simulink model "Main"  (R2025b)
settings: Solver=ode4  StartTime=0.0  StopTime=40  FixedStep=0.01  RelTol=1e-3
undefined symbols (not defined in the file): d_geo, DiscIntNeverNeededParam, t_geo, t_rotation, t_velocity
settings Model: DataDictionary=Main_data.sldd  VariantFading=off  Creator=mauro  LastModifiedBy=mauro

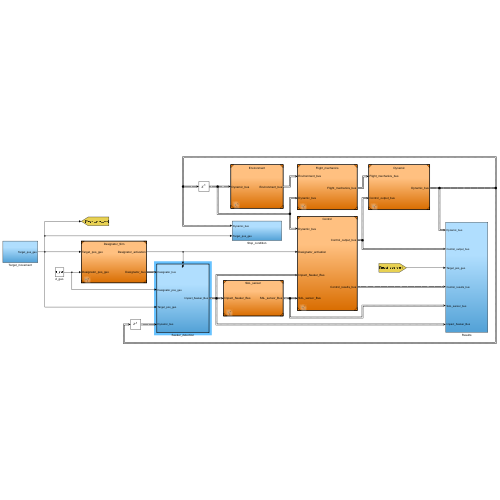
[thumbnail: Simulink's stored preview of the top-level diagram]
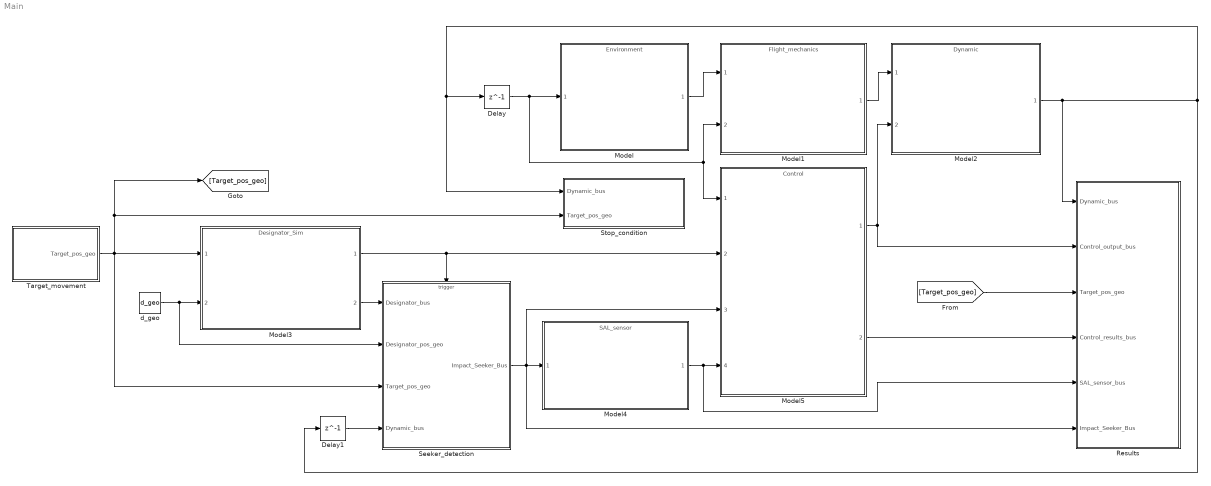
== system Main ==
  Delay : Delay  DelayLength=1  InitialCondition=0
  Delay1 : Delay  DelayLength=1  InitialCondition=0
  Model : ModelReference  ModelNameDialog=Environment.slx  SimulationMode=Normal  ModelReferenceVersion=1.30
  Model1 : ModelReference  ModelNameDialog=Flight_mechanics.slx  SimulationMode=Normal  ModelReferenceVersion=1.31
  Model2 : ModelReference  ModelNameDialog=Dynamic.slx  SimulationMode=Normal  ModelReferenceVersion=1.41
  Model3 : ModelReference  ModelNameDialog=Designator_Sim.slx  SimulationMode=Normal  ModelReferenceVersion=1.21
  Model4 : ModelReference  ModelNameDialog=SAL_sensor.slx  SimulationMode=Normal  ModelReferenceVersion=1.37
  Model5 : ModelReference  ModelNameDialog=Control.slx  SimulationMode=Normal  ModelReferenceVersion=1.50
  Results : Subsystem
  Seeker_detection : Subsystem
  Stop_condition : Subsystem
  Target_movement : Subsystem
  d_geo : Constant  Value=d_geo
  wires:
  Model1/1 -> Model2/1
  Model/1 -> Model1/1
  Model2/1 -> Delay1/1, Stop_condition/1(Dynamic_bus), Delay/1, Results/1(Dynamic_bus)
  Delay/1 -> Model5/1, Model1/2, Model/1
  Seeker_detection/1(Impact_Seeker_Bus) -> Model5/3, Results/6(Impact_Seeker_Bus), Model4/1
  Delay1/1 -> Seeker_detection/4(Dynamic_bus)
  Model3/2 -> Seeker_detection/1(Designator_bus)
  d_geo/1 -> Seeker_detection/2(Designator_pos_geo), Model3/2
  Model5/1 -> Results/2(Control_output_bus), Model2/2
  Model4/1 -> Results/5(SAL_sensor_bus), Model5/4
  Model3/1 -> Seeker_detection/Trigger, Model5/2
  [Target_pos_geo] -> Results/3(Target_pos_geo)
  Model5/2 -> Results/4(Control_results_bus)
  Target_movement/1(Target_pos_geo) -> Stop_condition/2(Target_pos_geo), [Target_pos_geo], Seeker_detection/3(Target_pos_geo), Model3/1

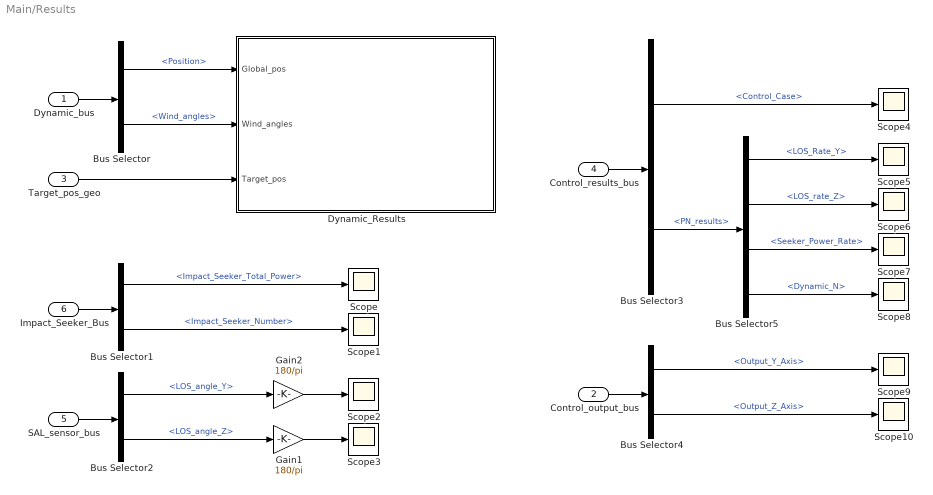
== system Main/Results ==
  Dynamic_bus : Inport  OutDataTypeStr=Bus: Dynamic_bus
  Control_output_bus : Inport  Port=2
  Target_pos_geo : Inport  Port=3
  Control_results_bus : Inport  Port=4
  SAL_sensor_bus : Inport  Port=5
  Impact_Seeker_Bus : Inport  Port=6
  Bus Selector : BusSelector  OutputSignals=Position,Wind_angles
  Bus Selector1 : BusSelector  OutputSignals=Impact_Seeker_Total_Power,Impact_Seeker_Number
  Bus Selector2 : BusSelector  OutputSignals=LOS_angle_Y,LOS_angle_Z
  Bus Selector3 : BusSelector  OutputSignals=Control_Case,PN_results
  Bus Selector4 : BusSelector  OutputSignals=Output_Y_Axis,Output_Z_Axis
  Bus Selector5 : BusSelector  OutputSignals=LOS_Rate_Y,LOS_rate_Z,Seeker_Power_Rate,Dynamic_N
  Dynamic_Results : Subsystem
  Gain1 : Gain  Gain=180/pi
  Gain2 : Gain  Gain=180/pi
  Scope{,1..10} (11 alike) : Scope
      Scope settings: ActiveDisplayYMinimum=-0.0017009499425087375  ActiveDisplayYMaximum=0.015308549482578641
      Scope1 settings: ActiveDisplayYMinimum=-4068.8424899316433  ActiveDisplayYMaximum=14541.688244827959  DataLoggingVariableName=ScopeData4
      Scope10 settings: ActiveDisplayYMinimum=-538.883824388517  ActiveDisplayYMaximum=718.00642075117651  DataLoggingVariableName=ScopeData13
      Scope2 settings: ActiveDisplayYMinimum=-1  ActiveDisplayYMaximum=1  DataLoggingVariableName=ScopeData5
      Scope3 settings: ActiveDisplayYMinimum=-9.0449990210259017  ActiveDisplayYMaximum=11.160194306089778  DataLoggingVariableName=ScopeData6
      Scope4 settings: ActiveDisplayYMinimum=-0.24999999999999994  ActiveDisplayYMaximum=2.25  DataLoggingVariableName=ScopeData7
      Scope5 settings: ActiveDisplayYMinimum=-0.00011873889811281793  ActiveDisplayYMaximum=0.00016852439541605621  DataLoggingVariableName=ScopeData8
      Scope6 settings: ActiveDisplayYMinimum=-0.65509945125026314  ActiveDisplayYMaximum=0.56583480808345421  DataLoggingVariableName=ScopeData9
      Scope7 settings: ActiveDisplayYMinimum=-0.26313284982804819  ActiveDisplayYMaximum=0.28806425796157659  DataLoggingVariableName=ScopeData10
      Scope8 settings: ActiveDisplayYMinimum=-0.25636599959653461  ActiveDisplayYMaximum=13.637920041276896  DataLoggingVariableName=ScopeData11
      Scope9 settings: ActiveDisplayYMinimum=-1  ActiveDisplayYMaximum=1  DataLoggingVariableName=ScopeData12
  wires:
  Dynamic_bus/1 -> Bus Selector/1
  Target_pos_geo/1 -> Dynamic_Results/3(Target_pos)
  Bus Selector/1 -> Dynamic_Results/1(Global_pos)  "<Position>"
  Bus Selector/2 -> Dynamic_Results/2(Wind_angles)  "<Wind_angles>"
  Impact_Seeker_Bus/1 -> Bus Selector1/1
  Bus Selector1/1 -> Scope/1  "<Impact_Seeker_Total_Power>"
  Bus Selector1/2 -> Scope1/1  "<Impact_Seeker_Number>"
  SAL_sensor_bus/1 -> Bus Selector2/1
  Bus Selector2/1 -> Gain2/1  "<LOS_angle_Y>"
  Bus Selector2/2 -> Gain1/1  "<LOS_angle_Z>"
  Control_results_bus/1 -> Bus Selector3/1
  Control_output_bus/1 -> Bus Selector4/1
  Bus Selector3/2 -> Bus Selector5/1  "<PN_results>"
  Bus Selector3/1 -> Scope4/1  "<Control_Case>"
  Bus Selector5/1 -> Scope5/1  "<LOS_Rate_Y>"
  Bus Selector5/2 -> Scope6/1  "<LOS_rate_Z>"
  Bus Selector5/4 -> Scope8/1  "<Dynamic_N>"
  Bus Selector5/3 -> Scope7/1  "<Seeker_Power_Rate>"
  Bus Selector4/1 -> Scope9/1  "<Output_Y_Axis>"
  Gain2/1 -> Scope2/1
  Gain1/1 -> Scope3/1
  Bus Selector4/2 -> Scope10/1  "<Output_Z_Axis>"

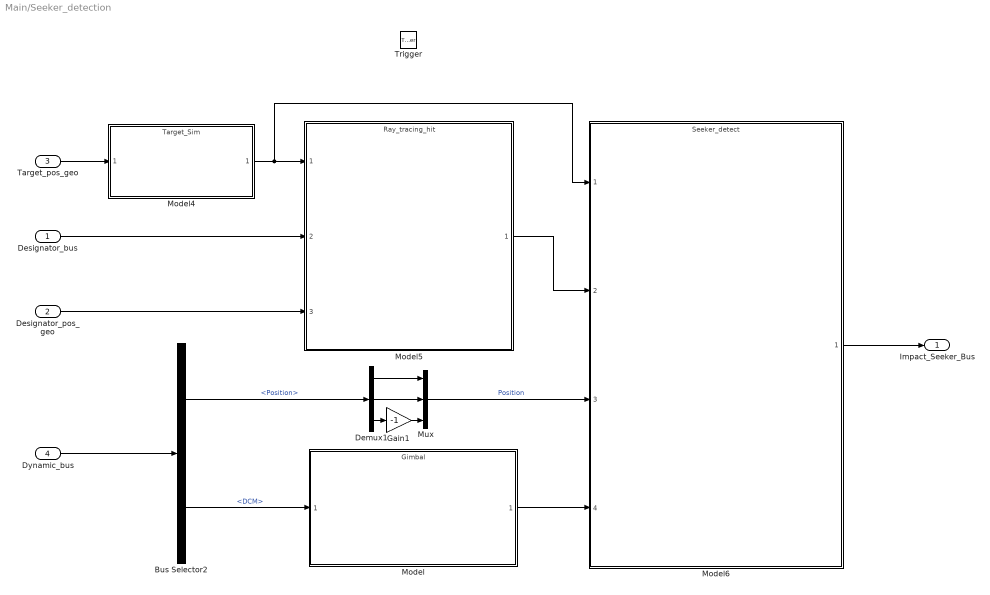
== system Main/Seeker_detection ==
  Designator_bus : Inport  OutDataTypeStr=Bus: Designator_bus
  Designator_pos_geo : Inport  Port=2
  Target_pos_geo : Inport  Port=3
  Dynamic_bus : Inport  Port=4  OutDataTypeStr=Bus: Dynamic_bus
  Trigger : TriggerPort  VariantControl=(inherit)  PortDimensions=1
  Bus Selector2 : BusSelector  OutputSignals=Position,DCM
  Demux1 : Demux  Outputs=3
  Gain1 : Gain  Gain=-1
  Model : ModelReference  ModelNameDialog=Gimbal.slx  SimulationMode=Normal  ModelReferenceVersion=1.16
  Model4 : ModelReference  ModelNameDialog=Target_Sim.slx  SimulationMode=Normal  ModelReferenceVersion=1.19
  Model5 : ModelReference  ModelNameDialog=Ray_tracing_hit.slx  SimulationMode=Normal  ModelReferenceVersion=1.26
  Model6 : ModelReference  ModelNameDialog=Seeker_detect.slx  SimulationMode=Normal  ModelReferenceVersion=1.23
  Mux : Mux  Inputs=3
  Impact_Seeker_Bus : Outport  OutDataTypeStr=Bus: Impact_Seeker_Bus
  wires:
  Model6/1 -> Impact_Seeker_Bus/1
  Model5/1 -> Model6/2
  Dynamic_bus/1 -> Bus Selector2/1
  Model4/1 -> Model6/1, Model5/1
  Target_pos_geo/1 -> Model4/1
  Designator_pos_geo/1 -> Model5/3
  Designator_bus/1 -> Model5/2
  Bus Selector2/1 -> Demux1/1  "<Position>"
  Bus Selector2/2 -> Model/1  "<DCM>"
  Model/1 -> Model6/4
  Demux1/1 -> Mux/1
  Demux1/3 -> Gain1/1
  Demux1/2 -> Mux/2
  Gain1/1 -> Mux/3
  Mux/1 -> Model6/3  "Position"

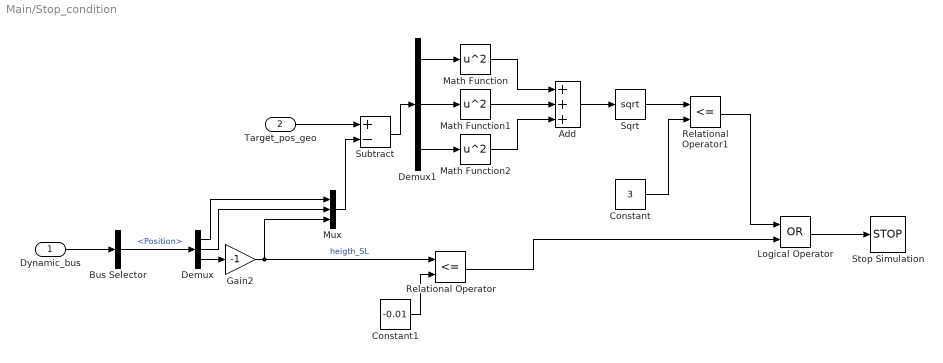
== system Main/Stop_condition ==
  Dynamic_bus : Inport  OutDataTypeStr=Bus: Dynamic_bus
  Target_pos_geo : Inport  Port=2
  Add : Sum  Inputs=+++
  Bus Selector : BusSelector  OutputSignals=Position
  Constant : Constant  Value=3
  Constant1 : Constant  Value=-0.01
  Demux : Demux  Outputs=3
  Demux1 : Demux  Outputs=3
  Gain2 : Gain  Gain=-1
  Logical Operator : Logic  Operator=OR  AllPortsSameDT=off  OutDataTypeStr=boolean
  Math Function : Math  Operator=square
  Math Function1 : Math  Operator=square
  Math Function2 : Math  Operator=square
  Mux : Mux  Inputs=3
  Relational Operator : RelationalOperator  Operator=<=  OutDataTypeStr=boolean  RndMeth=Simplest  InputSameDT=off
  Relational Operator1 : RelationalOperator  Operator=<=  OutDataTypeStr=boolean  RndMeth=Simplest  InputSameDT=off
  Sqrt : Sqrt
  Stop Simulation : Stop
  Subtract : Sum  Inputs=+-
  wires:
  Constant1/1 -> Relational Operator/2
  Dynamic_bus/1 -> Bus Selector/1
  Bus Selector/1 -> Demux/1  "<Position>"
  Demux/3 -> Gain2/1
  Gain2/1 -> Mux/3, Relational Operator/1  "heigth_SL"
  Logical Operator/1 -> Stop Simulation/1
  Relational Operator/1 -> Logical Operator/2
  Demux/1 -> Mux/1
  Demux/2 -> Mux/2
  Target_pos_geo/1 -> Subtract/1
  Mux/1 -> Subtract/2
  Subtract/1 -> Demux1/1
  Constant/1 -> Relational Operator1/2
  Demux1/1 -> Math Function/1
  Demux1/2 -> Math Function1/1
  Demux1/3 -> Math Function2/1
  Math Function1/1 -> Add/2
  Math Function/1 -> Add/1
  Math Function2/1 -> Add/3
  Add/1 -> Sqrt/1
  Sqrt/1 -> Relational Operator1/1
  Relational Operator1/1 -> Logical Operator/1

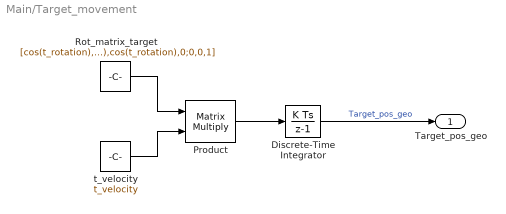
== system Main/Target_movement ==
  Discrete-Time Integrator : DiscreteIntegrator  InitialCondition=t_geo  SampleTime=-1  ICPrevOutput=DiscIntNeverNeededParam  ICPrevScaledInput=DiscIntNeverNeededParam
  Product : Product  Multiplication=Matrix(*)
  Rot_matrix_target : Constant  Value=[cos(t_rotation),-sin(t_rotation),0;sin(t_rotation),cos(t_rotation),0;0,0,1]
  t_velocity : Constant  Value=t_velocity
  Target_pos_geo : Outport
  wires:
  Rot_matrix_target/1 -> Product/1
  Product/1 -> Discrete-Time Integrator/1
  t_velocity/1 -> Product/2
  Discrete-Time Integrator/1 -> Target_pos_geo/1  "Target_pos_geo"

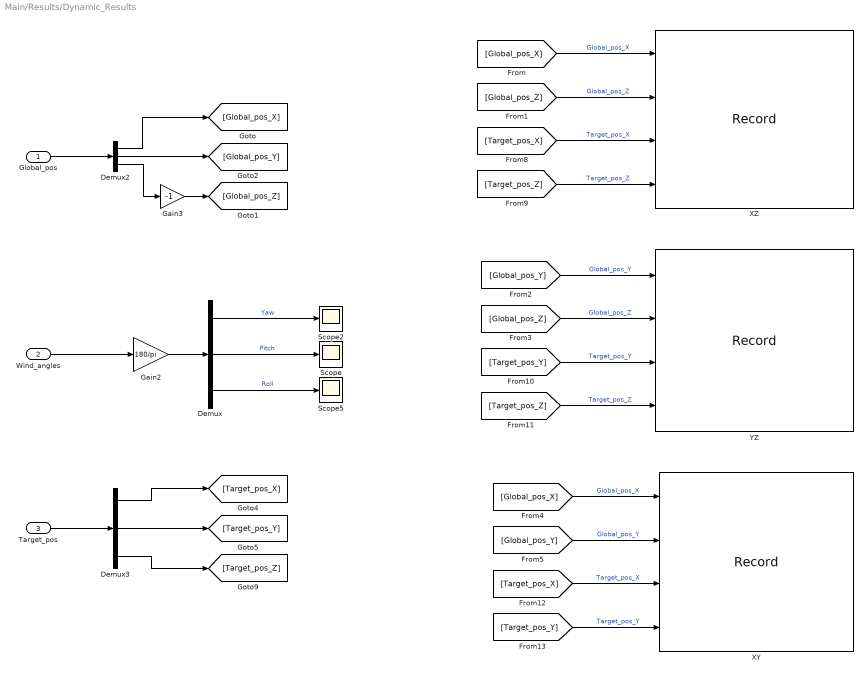
== system Main/Results/Dynamic_Results ==
  Global_pos : Inport
  Wind_angles : Inport  Port=2
  Target_pos : Inport  Port=3
  Demux : Demux  Outputs=3
  Demux2 : Demux  Outputs=3
  Demux3 : Demux  Outputs=3
  Gain2 : Gain  Gain=180/pi
  Gain3 : Gain  Gain=-1
  Scope : Scope
      settings: ActiveDisplayYMinimum=-31.267490052974193  ActiveDisplayYMaximum=20.037567055295582  DataLoggingVariableName=ScopeData2
  Scope2 : Scope
      settings: ActiveDisplayYMinimum=-76.139640294908645  ActiveDisplayYMaximum=235.78229244549729
  Scope5 : Scope
      settings: ActiveDisplayYMinimum=-22.500199563155505  ActiveDisplayYMaximum=202.50002217368396  DataLoggingVariableName=ScopeData3
  XY : Record  NumPorts=4.0  FileSettingsInternal="{\"entries\":[{\"content\":{\"excelSettings\":{\"content\":{},\"type\":\"Streamout.ExcelSettings\"},\"parquetSettings\":{\"content\":{},\"type\":\"Streamout.ParquetSettings\"}},\"type\":\"Streamout.FileSettingStorage\",\"uuid\":\"\"}],\"packageUris\":[\"http:\\/\\/schema.mathworks.com\\/mf0\\/streamout_blocks\\/R2020a\"],\"version\":\"1.0\"}"  FrameSettings=[0, 0, 0, 0]  Layout=[1 1]  SignalsInternal="{\"entries\":[{\"content\":{\"signals\":[{\"content\":{\"blockPath\":[],\"dimensions\":[1],\"domain\":\"\",\"lineColor\":\"#fe330a\",\"lineWidth\":2,\"plots\":[ 1 ],\"port\":1,\"sid\":[\"\"],\"signalID\":1,\"signalName\":\"Global_pos_X\"},\"type\":\"RecordBlkView.Signal\",\"uuid\":\"\"},{\"content\":{\"blockPath\":[],\"dimensions\":[1],\"domain\":\"\",\"lineColor\":\"#22b573\",\"lineWidth\":2,\"plots\":[ 1 ],\"port\":2,\"sid\":[\"\"],\"signalID\":2,\"signalName\":\"Global_pos_Y\"},\"type\":\"RecordBlkView.Signal\",\"uuid\":\"\"},{\"content\":{\"blockPath\":[],\"dimensions\":[1],\"domain\":\"\",\"lineColor\":\"#0072bd\",\"lineWidth\":2,\"plots\":[ 1 ],\"port\":3,\"sid\":[\"\"],\"signalID\":3,\"signalName\":\"Target_pos_X\"},\"type\":\"RecordBlkView.Signal\",\"uuid\":\"\"},{\"content\":{\"blockPath\":[],\"dimensions\":[1],\"domain\":\"\",\"lineColor\":\"#d95319\",\"lineWidth\":2,\"plots\":[ 1 ],\"port\":4,\"sid\":[\"\"],\"signalID\":4,\"signalName\":\"Target_pos_Y\"},\"type\":\"RecordBlkView.Signal\",\"uuid\":\"\"}]},\"type\":\"RecordBlkView.InputSignals\",\"uuid\":\"\"}],\"packageUris\":[\"http:\\/\\/schema.mathworks.com\\/mf0\\/streamout_blocks\\/R2020a\"],\"version\":\"1.0\"}"  VisualizationBindings="{\"xyplotplugin\":{\"info\":[{\"series\":[{\"bindingParametersList\":[{\"parameter\":\"X-Axis\",\"signalID\":1,\"signalName\":\"Global_pos_X\"},{\"parameter\":\"Y-Axis\",\"signalID\":2,\"signalName\":\"Global_pos_Y\"}],\"seriesID\":0},{\"bindingParametersList\":[{\"parameter\":\"X-Axis\",\"signalID\":3,\"signalName\":\"Target_pos_X\"},{\"parameter\":\"Y-Axis\",\"signalID\":4,\"signalName\":\"Target_pos_Y\"}],\"seriesID\":1}],\"subplotID\":1}]}}"  CompatibilityTag=XY
  XZ : Record  NumPorts=4.0  RecordToFile=on  FileSettingsInternal="{\"entries\":[{\"content\":{\"excelSettings\":{\"content\":{},\"type\":\"Streamout.ExcelSettings\"},\"parquetSettings\":{\"content\":{},\"type\":\"Streamout.ParquetSettings\"}},\"type\":\"Streamout.FileSettingStorage\",\"uuid\":\"\"}],\"packageUris\":[\"http:\\/\\/schema.mathworks.com\\/mf0\\/streamout_blocks\\/R2020a\"],\"version\":\"1.0\"}"  FrameSettings=[0, 0, 0, 0]  Layout=[1 1]  SignalsInternal="{\"entries\":[{\"content\":{\"signals\":[{\"content\":{\"blockPath\":[],\"dimensions\":[1],\"domain\":\"\",\"lineColor\":\"#d95319\",\"lineWidth\":2,\"plots\":[ 1 ],\"port\":1,\"sid\":[\"\"],\"signalID\":1,\"signalName\":\"Global_pos_X\"},\"type\":\"RecordBlkView.Signal\",\"uuid\":\"\"},{\"content\":{\"blockPath\":[],\"dimensions\":[1],\"domain\":\"\",\"lineColor\":\"#edb120\",\"lineWidth\":2,\"plots\":[ 1 ],\"port\":2,\"sid\":[\"\"],\"signalID\":2,\"signalName\":\"Global_pos_Z\"},\"type\":\"RecordBlkView.Signal\",\"uuid\":\"\"},{\"content\":{\"blockPath\":[],\"dimensions\":[1],\"domain\":\"\",\"lineColor\":\"#7e2f8e\",\"lineWidth\":2,\"plots\":[ 1 ],\"port\":3,\"sid\":[\"\"],\"signalID\":3,\"signalName\":\"Target_pos_X\"},\"type\":\"RecordBlkView.Signal\",\"uuid\":\"\"},{\"content\":{\"blockPath\":[],\"dimensions\":[1],\"domain\":\"\",\"lineColor\":\"#77ac30\",\"lineWidth\":2,\"plots\":[ 1 ],\"port\":4,\"sid\":[\"\"],\"signalID\":4,\"signalName\":\"Target_pos_Z\"},\"type\":\"RecordBlkView.Signal\",\"uuid\":\"\"}]},\"type\":\"RecordBlkView.InputSignals\",\"uuid\":\"\"}],\"packageUris\":[\"http:\\/\\/schema.mathworks.com\\/mf0\\/streamout_blocks\\/R2020a\"],\"version\":\"1.0\"}"  VisualizationBindings="{\"xyplotplugin\":{\"info\":[{\"series\":[{\"bindingParametersList\":[{\"parameter\":\"X-Axis\",\"signalID\":1,\"signalName\":\"Global_pos_X\"},{\"parameter\":\"Y-Axis\",\"signalID\":2,\"signalName\":\"Global_pos_Z\"}],\"seriesID\":0},{\"bindingParametersList\":[{\"parameter\":\"X-Axis\",\"signalID\":3,\"signalName\":\"Target_pos_X\"},{\"parameter\":\"Y-Axis\",\"signalID\":4,\"signalName\":\"Target_pos_Z\"}],\"seriesID\":1}],\"subplotID\":1}]}}"  CompatibilityTag=XY
  YZ : Record  NumPorts=4.0  FileSettingsInternal="{\"entries\":[{\"content\":{\"excelSettings\":{\"content\":{},\"type\":\"Streamout.ExcelSettings\"},\"parquetSettings\":{\"content\":{},\"type\":\"Streamout.ParquetSettings\"}},\"type\":\"Streamout.FileSettingStorage\",\"uuid\":\"\"}],\"packageUris\":[\"http:\\/\\/schema.mathworks.com\\/mf0\\/streamout_blocks\\/R2020a\"],\"version\":\"1.0\"}"  FrameSettings=[0, 0, 0, 0]  Layout=[1 1]  SignalsInternal="{\"entries\":[{\"content\":{\"signals\":[{\"content\":{\"blockPath\":[],\"dimensions\":[1],\"domain\":\"\",\"lineColor\":\"#a2142f\",\"lineWidth\":2,\"port\":1,\"sid\":[\"\"],\"signalID\":1,\"signalName\":\"Global_pos_Y\"},\"type\":\"RecordBlkView.Signal\",\"uuid\":\"\"},{\"content\":{\"blockPath\":[],\"dimensions\":[1],\"domain\":\"\",\"lineColor\":\"#139fff\",\"lineWidth\":2,\"port\":2,\"sid\":[\"\"],\"signalID\":2,\"signalName\":\"Global_pos_Z\"},\"type\":\"RecordBlkView.Signal\",\"uuid\":\"\"},{\"content\":{\"blockPath\":[],\"dimensions\":[1],\"domain\":\"\",\"lineColor\":\"#ff6929\",\"lineWidth\":2,\"port\":3,\"sid\":[\"\"],\"signalID\":3,\"signalName\":\"Target_pos_Y\"},\"type\":\"RecordBlkView.Signal\",\"uuid\":\"\"},{\"content\":{\"blockPath\":[],\"dimensions\":[1],\"domain\":\"\",\"lineColor\":\"#b746ff\",\"lineWidth\":2,\"port\":4,\"sid\":[\"\"],\"signalID\":4,\"signalName\":\"Target_pos_Z\"},\"type\":\"RecordBlkView.Signal\",\"uuid\":\"\"}]},\"type\":\"RecordBlkView.InputSignals\",\"uuid\":\"\"}],\"packageUris\":[\"http:\\/\\/schema.mathworks.com\\/mf0\\/streamout_blocks\\/R2020a\"],\"version\":\"1.0\"}"  VisualizationBindings="{\"xyplotplugin\":{\"info\":[{\"series\":[],\"subplotID\":1}]}}"  CompatibilityTag=XY
  wires:
  Gain2/1 -> Demux/1
  [Global_pos_Y] -> YZ/1  "Global_pos_Y"
  Demux/2 -> Scope/1  "Pitch"
  Demux/1 -> Scope2/1  "Yaw"
  Demux/3 -> Scope5/1  "Roll"
  [Target_pos_Y] -> YZ/3  "Target_pos_Y"
  [Global_pos_Z] -> XZ/2  "Global_pos_Z"
  [Target_pos_Z] -> YZ/4  "Target_pos_Z"
  Demux2/1 -> [Global_pos_X]
  Demux3/2 -> [Target_pos_Y]
  [Global_pos_Z] -> YZ/2  "Global_pos_Z"
  [Target_pos_X] -> XY/3  "Target_pos_X"
  [Target_pos_Y] -> XY/4  "Target_pos_Y"
  [Target_pos_Z] -> XZ/4  "Target_pos_Z"
  Demux2/2 -> [Global_pos_Y]
  [Global_pos_X] -> XY/1  "Global_pos_X"
  [Global_pos_Y] -> XY/2  "Global_pos_Y"
  [Global_pos_X] -> XZ/1  "Global_pos_X"
  Demux2/3 -> Gain3/1
  [Target_pos_X] -> XZ/3  "Target_pos_X"
  Demux3/3 -> [Target_pos_Z]
  Demux3/1 -> [Target_pos_X]
  Wind_angles/1 -> Gain2/1
  Gain3/1 -> [Global_pos_Z]
  Target_pos/1 -> Demux3/1
  Global_pos/1 -> Demux2/1
